simulink model "Pipe_Geometry_1"  (Simulink 7.6)
settings: Solver=ode45  StartTime=0.0  StopTime=3600  RelTol=1e-5
settings Model: Creator=drhf  LastModifiedBy=awohlfei
settings CodeAppCC: CustomSymbolStrType=$N$R$M_T

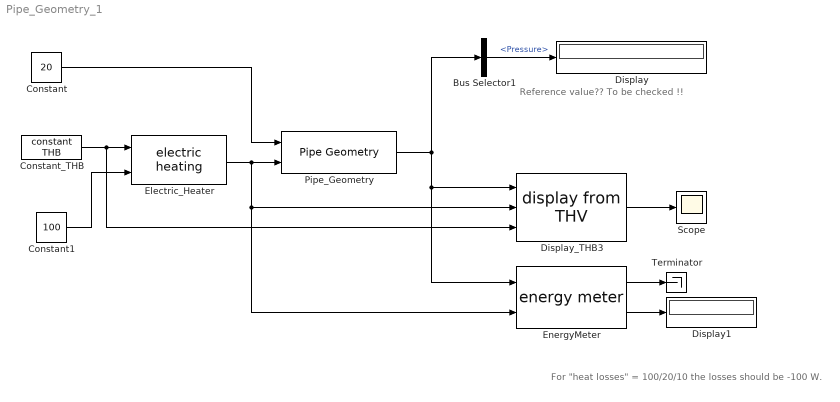
== system Pipe_Geometry_1 ==
  note: For "heat losses" = 100/20/10
      | the losses should be -100 W.
  note: Reference value??
      | To be checked !!
  Bus Selector1 : BusSelector  OutputSignals=Pressure
  Constant : Constant  Value=20
  Constant1 : Constant  Value=100
  Constant_THB : Reference  SystemSampleTime=-1  t=40  mdot=720/3600  p=1e5  mID=Full Pressure Drop with Static Height  fluid=water  mix=0  dia=10  hgt=0
  Display : Display
      settings: Format=decimal (Stored Integer)
  Display1 : Display
  Display_THB3 : Reference  SystemSampleTime=-1  t=on  m=off  p=off  id=off  mix=off  d=off
  Electric_Heater : Reference  SystemSampleTime=-1
  EnergyMeter : Reference  SystemSampleTime=-1
  Pipe_Geometry : Reference  SystemSampleTime=-1  dia=0.02  len=10  hgt=0  uloss=100/20/10  cond=0  cwall=1000  t0=20  rough=0.04*1e-3  nbend=4  nodes=1
  Scope : Scope
      settings: TimeRange=4000  YMin=39.66951326595616  YMax=40.42277164649369
  Terminator : Terminator
  wires:
  Constant/1 -> Pipe_Geometry/1
  Pipe_Geometry/1 -> Bus Selector1/1, Display_THB3/1, EnergyMeter/1
  Bus Selector1/1 -> Display/1  "<Pressure>"
  Constant_THB/1 -> Electric_Heater/1, Display_THB3/3
  Electric_Heater/1 -> Display_THB3/2, EnergyMeter/2, Pipe_Geometry/2
  Constant1/1 -> Electric_Heater/2
  Display_THB3/1 -> Scope/1
  EnergyMeter/2 -> Display1/1
  EnergyMeter/1 -> Terminator/1
